simulink library "inp"  (R2021b)
settings: Solver=VariableStepAuto  StartTime=0.0  StopTime=10.0  RelTol=1e-3
undefined symbols (not defined in the file): C_TASK_5MS_S, FALSE, KINP_AcoreReadyToSlp_flg_ovrdflg, KINP_AcoreReadyToSlp_flg_ovrdval, KINP_AllowMovThd_OTA_enum_ovrdflg, KINP_AllowMovThd_OTA_enum_ovrdval, KINP_APSAngleTarget_Deg_ovrdflg, KINP_APSAngleTarget_Deg_ovrdval, KINP_APSDecReq_mps2_ovrdflg, KINP_APSDecReq_mps2_ovrdval, KINP_APSDecReqA_flg_ovrdflg, KINP_APSDecReqA_flg_ovrdval, KINP_APSDFLL_cm_ovrdflg, KINP_APSDFLL_cm_ovrdval, KINP_APSDFLR_cm_ovrdflg, KINP_APSDFLR_cm_ovrdval, KINP_APSDRLL_cm_ovrdflg, KINP_APSDRLL_cm_ovrdval, KINP_APSDRLR_cm_ovrdflg, KINP_APSDRLR_cm_ovrdval, KINP_APSExitCondition_enum_ovrdflg, KINP_APSExitCondition_enum_ovrdval, KINP_APSHWVer_enum_ovrdflg, KINP_APSHWVer_enum_ovrdval, KINP_APSProgressPCT_pct_ovrdflg, KINP_APSProgressPCT_pct_ovrdval, KINP_APSReq_enum_ovrdflg, KINP_APSReq_enum_ovrdval, KINP_APSRQDisplay_enum_ovrdflg, KINP_APSRQDisplay_enum_ovrdval, KINP_APSRqEPASCtrl_flg_ovrdflg, KINP_APSRqEPASCtrl_flg_ovrdval, KINP_APSShiftPosnReq_enum_ovrdval, KINP_APSShiftPosnReq_enum_ovrflg, KINP_APSSpeedCMD_kph_ovrdval, KINP_APSSpeedCMD_kph_ovrflg, KINP_APSStaSystem_enum_ovrdflg, KINP_APSStaSystem_enum_ovrdval, KINP_APSSWVer_enum_ovrdflg, KINP_APSSWVer_enum_ovrdval, KINP_APSVMCReqA_flg_ovrdval, KINP_APSVMCReqA_flg_ovrflg, KINP_APSVRqEPASCtrl_flg_ovrdflg, KINP_APSVRqEPASCtrl_flg_ovrdval, KINP_AuxBattVolmV_mV_ovrdflg, KINP_AuxBattVolmV_mV_ovrdval, KINP_CAASSta_enum_ovrdflg, KINP_CAASSta_enum_ovrdval, KINP_CAASVMCReqA_flg_ovrdval, KINP_CAASVMCReqA_flg_ovrflg, KINP_Chime_enum_ovrdflg, KINP_Chime_enum_ovrdval, KINP_ClearDTCcmd_flg_ovrdflg, KINP_ClearDTCcmd_flg_ovrdval, KINP_EvccAplusPwrUpReq_flg_ovrdflg, KINP_EvccAplusPwrUpReq_flg_ovrdval, KINP_LFID_raw_ovrdval, KINP_LFID_raw_ovrflg, KINP_LRID_raw_ovrdval, KINP_MemOffsetAccX_raw16_ovrdflg ... (+118)
libraries: FVT_lib x595, hcu_lib x1
(part 20 of 27)

== system inp/INP/CAN3/SignalCheck/MCU_F2 ==
  BHAL_outputs : Inport
  inp_CanValid_bus : Inport  Port=2
  FrCoolanttempReq : FVT_lib/inp/can_signal_template  SystemSampleTime=-1  VariantActivationTime=update diagram  Latency=0  AutoFrameSizeCalculation=off
      link override defval: Value=KINP_FrCoolanttempReq_C_defval
      link override fftdec: Value=KINP_FrCoolanttempReq_C_fftdec
      link override fftinc: Value=KINP_FrCoolanttempReq_C_fftinc
      link override fftlim: Value=KINP_FrCoolanttempReq_C_fftlim
      link override invalid: Value=KINP_FrCoolanttempReq_C_invalid
      link override ovrdflg: Value=KINP_FrCoolanttempReq_C_ovrdflg
      link override ovrdval: Value=KINP_FrCoolanttempReq_C_ovrdval
      link override setvalid: Value=KINP_FrCoolanttempReq_C_setvalid
      link override srvcflg: Value=KINP_FrCoolanttempReq_C_srvcflg
      link override srvcval: Value=KINP_FrCoolanttempReq_C_srvcval
  FrEOPSpdSet : FVT_lib/inp/can_signal_template  SystemSampleTime=-1  VariantActivationTime=update diagram  Latency=0  AutoFrameSizeCalculation=off
      link override defval: Value=KINP_FrEOPSpdSet_rpm_defval
      link override fftdec: Value=KINP_FrEOPSpdSet_rpm_fftdec
      link override fftinc: Value=KINP_FrEOPSpdSet_rpm_fftinc
      link override fftlim: Value=KINP_FrEOPSpdSet_rpm_fftlim
      link override invalid: Value=KINP_FrEOPSpdSet_rpm_invalid
      link override ovrdflg: Value=KINP_FrEOPSpdSet_rpm_ovrdflg
      link override ovrdval: Value=KINP_FrEOPSpdSet_rpm_ovrdval
      link override setvalid: Value=KINP_FrEOPSpdSet_rpm_setvalid
      link override srvcflg: Value=KINP_FrEOPSpdSet_rpm_srvcflg
      link override srvcval: Value=KINP_FrEOPSpdSet_rpm_srvcval
  FrFailcode1 : FVT_lib/inp/can_signal_template  SystemSampleTime=-1  VariantActivationTime=update diagram  Latency=0  AutoFrameSizeCalculation=off
      link override defval: Value=KINP_FrFailcode1_enum_defval
      link override fftdec: Value=KINP_FrFailcode1_enum_fftdec
      link override fftinc: Value=KINP_FrFailcode1_enum_fftinc
      link override fftlim: Value=KINP_FrFailcode1_enum_fftlim
      link override invalid: Value=KINP_FrFailcode1_enum_invalid
      link override ovrdflg: Value=KINP_FrFailcode1_enum_ovrdflg
      link override ovrdval: Value=KINP_FrFailcode1_enum_ovrdval
      link override setvalid: Value=KINP_FrFailcode1_enum_setvalid
      link override srvcflg: Value=KINP_FrFailcode1_enum_srvcflg
      link override srvcval: Value=KINP_FrFailcode1_enum_srvcval
  FrFailcode2 : FVT_lib/inp/can_signal_template  SystemSampleTime=-1  VariantActivationTime=update diagram  Latency=0  AutoFrameSizeCalculation=off
      link override defval: Value=KINP_FrFailcode2_enum_defval
      link override fftdec: Value=KINP_FrFailcode2_enum_fftdec
      link override fftinc: Value=KINP_FrFailcode2_enum_fftinc
      link override fftlim: Value=KINP_FrFailcode2_enum_fftlim
      link override invalid: Value=KINP_FrFailcode2_enum_invalid
      link override ovrdflg: Value=KINP_FrFailcode2_enum_ovrdflg
      link override ovrdval: Value=KINP_FrFailcode2_enum_ovrdval
      link override setvalid: Value=KINP_FrFailcode2_enum_setvalid
      link override srvcflg: Value=KINP_FrFailcode2_enum_srvcflg
      link override srvcval: Value=KINP_FrFailcode2_enum_srvcval
  FrFailcodehistory1 : FVT_lib/inp/can_signal_template  SystemSampleTime=-1  VariantActivationTime=update diagram  Latency=0  AutoFrameSizeCalculation=off
      link override defval: Value=KINP_FrFailcodehistory1_enum_defval
      link override fftdec: Value=KINP_FrFailcodehistory1_enum_fftdec
      link override fftinc: Value=KINP_FrFailcodehistory1_enum_fftinc
      link override fftlim: Value=KINP_FrFailcodehistory1_enum_fftlim
      link override invalid: Value=KINP_FrFailcodehistory1_enum_invalid
      link override ovrdflg: Value=KINP_FrFailcodehistory1_enum_ovrdflg
      link override ovrdval: Value=KINP_FrFailcodehistory1_enum_ovrdval
      link override setvalid: Value=KINP_FrFailcodehistory1_enum_setvalid
      link override srvcflg: Value=KINP_FrFailcodehistory1_enum_srvcflg
      link override srvcval: Value=KINP_FrFailcodehistory1_enum_srvcval
  FrFailcodehistory2 : FVT_lib/inp/can_signal_template  SystemSampleTime=-1  VariantActivationTime=update diagram  Latency=0  AutoFrameSizeCalculation=off
      link override defval: Value=KINP_FrFailcodehistory2_enum_defval
      link override fftdec: Value=KINP_FrFailcodehistory2_enum_fftdec
      link override fftinc: Value=KINP_FrFailcodehistory2_enum_fftinc
      link override fftlim: Value=KINP_FrFailcodehistory2_enum_fftlim
      link override invalid: Value=KINP_FrFailcodehistory2_enum_invalid
      link override ovrdflg: Value=KINP_FrFailcodehistory2_enum_ovrdflg
      link override ovrdval: Value=KINP_FrFailcodehistory2_enum_ovrdval
      link override setvalid: Value=KINP_FrFailcodehistory2_enum_setvalid
      link override srvcflg: Value=KINP_FrFailcodehistory2_enum_srvcflg
      link override srvcval: Value=KINP_FrFailcodehistory2_enum_srvcval
  FrLLCTemp : FVT_lib/inp/can_signal_template  SystemSampleTime=-1  VariantActivationTime=update diagram  Latency=0  AutoFrameSizeCalculation=off
      link override defval: Value=KINP_FrLLCTemp_C_defval
      link override fftdec: Value=KINP_FrLLCTemp_C_fftdec
      link override fftinc: Value=KINP_FrLLCTemp_C_fftinc
      link override fftlim: Value=KINP_FrLLCTemp_C_fftlim
      link override invalid: Value=KINP_FrLLCTemp_C_invalid
      link override ovrdflg: Value=KINP_FrLLCTemp_C_ovrdflg
      link override ovrdval: Value=KINP_FrLLCTemp_C_ovrdval
      link override setvalid: Value=KINP_FrLLCTemp_C_setvalid
      link override srvcflg: Value=KINP_FrLLCTemp_C_srvcflg
      link override srvcval: Value=KINP_FrLLCTemp_C_srvcval
  FrLLCflowReq : FVT_lib/inp/can_signal_template  SystemSampleTime=-1  VariantActivationTime=update diagram  Latency=0  AutoFrameSizeCalculation=off
      link override defval: Value=KINP_FrLLCflowReq_Lpmin_defval
      link override fftdec: Value=KINP_FrLLCflowReq_Lpmin_fftdec
      link override fftinc: Value=KINP_FrLLCflowReq_Lpmin_fftinc
      link override fftlim: Value=KINP_FrLLCflowReq_Lpmin_fftlim
      link override invalid: Value=KINP_FrLLCflowReq_Lpmin_invalid
      link override ovrdflg: Value=KINP_FrLLCflowReq_Lpmin_ovrdflg
      link override ovrdval: Value=KINP_FrLLCflowReq_Lpmin_ovrdval
      link override setvalid: Value=KINP_FrLLCflowReq_Lpmin_setvalid
      link override srvcflg: Value=KINP_FrLLCflowReq_Lpmin_srvcflg
      link override srvcval: Value=KINP_FrLLCflowReq_Lpmin_srvcval
  FrMCUTempWarn : FVT_lib/inp/can_signal_template  SystemSampleTime=-1  VariantActivationTime=update diagram  Latency=0  AutoFrameSizeCalculation=off
      link override defval: Value=KINP_FrMCUTempWarn_enum_defval
      link override fftdec: Value=KINP_FrMCUTempWarn_enum_fftdec
      link override fftinc: Value=KINP_FrMCUTempWarn_enum_fftinc
      link override fftlim: Value=KINP_FrMCUTempWarn_enum_fftlim
      link override invalid: Value=KINP_FrMCUTempWarn_enum_invalid
      link override ovrdflg: Value=KINP_FrMCUTempWarn_enum_ovrdflg
      link override ovrdval: Value=KINP_FrMCUTempWarn_enum_ovrdval
      link override setvalid: Value=KINP_FrMCUTempWarn_enum_setvalid
      link override srvcflg: Value=KINP_FrMCUTempWarn_enum_srvcflg
      link override srvcval: Value=KINP_FrMCUTempWarn_enum_srvcval
  FrTMTempWarn : FVT_lib/inp/can_signal_template  SystemSampleTime=-1  VariantActivationTime=update diagram  Latency=0  AutoFrameSizeCalculation=off
      link override defval: Value=KINP_FrTMTempWarn_enum_defval
      link override fftdec: Value=KINP_FrTMTempWarn_enum_fftdec
      link override fftinc: Value=KINP_FrTMTempWarn_enum_fftinc
      link override fftlim: Value=KINP_FrTMTempWarn_enum_fftlim
      link override invalid: Value=KINP_FrTMTempWarn_enum_invalid
      link override ovrdflg: Value=KINP_FrTMTempWarn_enum_ovrdflg
      link override ovrdval: Value=KINP_FrTMTempWarn_enum_ovrdval
      link override setvalid: Value=KINP_FrTMTempWarn_enum_setvalid
      link override srvcflg: Value=KINP_FrTMTempWarn_enum_srvcflg
      link override srvcval: Value=KINP_FrTMTempWarn_enum_srvcval
  Terminator_{1..10} (10 alike) : Terminator
  True_VHAL_FrCoolanttempReq_C : Constant  Value=TRUE  OutDataTypeStr=boolean
  True_VHAL_FrEOPSpdSet_rpm : Constant  Value=TRUE  OutDataTypeStr=boolean
  True_VHAL_FrFailcode1_enum : Constant  Value=TRUE  OutDataTypeStr=boolean
  True_VHAL_FrFailcode2_enum : Constant  Value=TRUE  OutDataTypeStr=boolean
  True_VHAL_FrFailcodehistory1_enum : Constant  Value=TRUE  OutDataTypeStr=boolean
  True_VHAL_FrFailcodehistory2_enum : Constant  Value=TRUE  OutDataTypeStr=boolean
  True_VHAL_FrLLCTemp_C : Constant  Value=TRUE  OutDataTypeStr=boolean
  True_VHAL_FrLLCflowReq_Lpmin : Constant  Value=TRUE  OutDataTypeStr=boolean
  True_VHAL_FrMCUTempWarn_enum : Constant  Value=TRUE  OutDataTypeStr=boolean
  True_VHAL_FrTMTempWarn_enum : Constant  Value=TRUE  OutDataTypeStr=boolean
  slr1_{1..10} (10 alike) : BusSelector  OutputSignals=VINP_CANMsgValidMCUF2_flg
  slr_VHAL_FrCoolanttempReq_C : BusSelector  OutputSignals=VHAL_FrCoolanttempReq_C
  slr_VHAL_FrEOPSpdSet_rpm : BusSelector  OutputSignals=VHAL_FrEOPSpdSet_rpm
  slr_VHAL_FrFailcode1_enum : BusSelector  OutputSignals=VHAL_FrFailcode1_enum
  slr_VHAL_FrFailcode2_enum : BusSelector  OutputSignals=VHAL_FrFailcode2_enum
  slr_VHAL_FrFailcodehistory1_enum : BusSelector  OutputSignals=VHAL_FrFailcodehistory1_enum
  slr_VHAL_FrFailcodehistory2_enum : BusSelector  OutputSignals=VHAL_FrFailcodehistory2_enum
  slr_VHAL_FrLLCTemp_C : BusSelector  OutputSignals=VHAL_FrLLCTemp_C
  slr_VHAL_FrLLCflowReq_Lpmin : BusSelector  OutputSignals=VHAL_FrLLCflowReq_Lpmin
  slr_VHAL_FrMCUTempWarn_enum : BusSelector  OutputSignals=VHAL_FrMCUTempWarn_enum
  slr_VHAL_FrTMTempWarn_enum : BusSelector  OutputSignals=VHAL_FrTMTempWarn_enum
  VINP_FrCoolanttempReq_C : Outport
  VINP_FrEOPSpdSet_rpm : Outport  Port=2
  VINP_FrFailcode1_enum : Outport  Port=3
  VINP_FrFailcode2_enum : Outport  Port=4
  VINP_FrFailcodehistory1_enum : Outport  Port=5
  VINP_FrFailcodehistory2_enum : Outport  Port=6
  VINP_FrLLCTemp_C : Outport  Port=7
  VINP_FrLLCflowReq_Lpmin : Outport  Port=8
  VINP_FrMCUTempWarn_enum : Outport  Port=9
  VINP_FrTMTempWarn_enum : Outport  Port=10
  wires:
  BHAL_outputs/1 -> [BHAL_outputs]
  inp_CanValid_bus/1 -> [inp_CanValid_bus]
  [BHAL_outputs] -> slr_VHAL_FrCoolanttempReq_C/1
  slr_VHAL_FrCoolanttempReq_C/1 -> FrCoolanttempReq/1  "<VHAL_FrCoolanttempReq_C>"
  True_VHAL_FrCoolanttempReq_C/1 -> FrCoolanttempReq/2
  [inp_CanValid_bus] -> slr1_1/1
  slr1_1/1 -> FrCoolanttempReq/3  "<VINP_CANMsgValidMCUF2_flg>"
  FrCoolanttempReq/1 -> VINP_FrCoolanttempReq_C/1  "VINP_FrCoolanttempReq_C"
  FrCoolanttempReq/2 -> Terminator_1/1
  [BHAL_outputs] -> slr_VHAL_FrEOPSpdSet_rpm/1
  slr_VHAL_FrEOPSpdSet_rpm/1 -> FrEOPSpdSet/1  "<VHAL_FrEOPSpdSet_rpm>"
  True_VHAL_FrEOPSpdSet_rpm/1 -> FrEOPSpdSet/2
  [inp_CanValid_bus] -> slr1_2/1
  slr1_2/1 -> FrEOPSpdSet/3  "<VINP_CANMsgValidMCUF2_flg>"
  FrEOPSpdSet/1 -> VINP_FrEOPSpdSet_rpm/1  "VINP_FrEOPSpdSet_rpm"
  FrEOPSpdSet/2 -> Terminator_2/1
  [BHAL_outputs] -> slr_VHAL_FrFailcode1_enum/1
  slr_VHAL_FrFailcode1_enum/1 -> FrFailcode1/1  "<VHAL_FrFailcode1_enum>"
  True_VHAL_FrFailcode1_enum/1 -> FrFailcode1/2
  [inp_CanValid_bus] -> slr1_3/1
  slr1_3/1 -> FrFailcode1/3  "<VINP_CANMsgValidMCUF2_flg>"
  FrFailcode1/1 -> VINP_FrFailcode1_enum/1  "VINP_FrFailcode1_enum"
  FrFailcode1/2 -> Terminator_3/1
  [BHAL_outputs] -> slr_VHAL_FrFailcode2_enum/1
  slr_VHAL_FrFailcode2_enum/1 -> FrFailcode2/1  "<VHAL_FrFailcode2_enum>"
  True_VHAL_FrFailcode2_enum/1 -> FrFailcode2/2
  [inp_CanValid_bus] -> slr1_4/1
  slr1_4/1 -> FrFailcode2/3  "<VINP_CANMsgValidMCUF2_flg>"
  FrFailcode2/1 -> VINP_FrFailcode2_enum/1  "VINP_FrFailcode2_enum"
  FrFailcode2/2 -> Terminator_4/1
  [BHAL_outputs] -> slr_VHAL_FrFailcodehistory1_enum/1
  slr_VHAL_FrFailcodehistory1_enum/1 -> FrFailcodehistory1/1  "<VHAL_FrFailcodehistory1_enum>"
  True_VHAL_FrFailcodehistory1_enum/1 -> FrFailcodehistory1/2
  [inp_CanValid_bus] -> slr1_5/1
  slr1_5/1 -> FrFailcodehistory1/3  "<VINP_CANMsgValidMCUF2_flg>"
  FrFailcodehistory1/1 -> VINP_FrFailcodehistory1_enum/1  "VINP_FrFailcodehistory1_enum"
  FrFailcodehistory1/2 -> Terminator_5/1
  [BHAL_outputs] -> slr_VHAL_FrFailcodehistory2_enum/1
  slr_VHAL_FrFailcodehistory2_enum/1 -> FrFailcodehistory2/1  "<VHAL_FrFailcodehistory2_enum>"
  True_VHAL_FrFailcodehistory2_enum/1 -> FrFailcodehistory2/2
  [inp_CanValid_bus] -> slr1_6/1
  slr1_6/1 -> FrFailcodehistory2/3  "<VINP_CANMsgValidMCUF2_flg>"
  FrFailcodehistory2/1 -> VINP_FrFailcodehistory2_enum/1  "VINP_FrFailcodehistory2_enum"
  FrFailcodehistory2/2 -> Terminator_6/1
  [BHAL_outputs] -> slr_VHAL_FrLLCTemp_C/1
  slr_VHAL_FrLLCTemp_C/1 -> FrLLCTemp/1  "<VHAL_FrLLCTemp_C>"
  True_VHAL_FrLLCTemp_C/1 -> FrLLCTemp/2
  [inp_CanValid_bus] -> slr1_7/1
  slr1_7/1 -> FrLLCTemp/3  "<VINP_CANMsgValidMCUF2_flg>"
  FrLLCTemp/1 -> VINP_FrLLCTemp_C/1  "VINP_FrLLCTemp_C"
  FrLLCTemp/2 -> Terminator_7/1
  [BHAL_outputs] -> slr_VHAL_FrLLCflowReq_Lpmin/1
  slr_VHAL_FrLLCflowReq_Lpmin/1 -> FrLLCflowReq/1  "<VHAL_FrLLCflowReq_Lpmin>"
  True_VHAL_FrLLCflowReq_Lpmin/1 -> FrLLCflowReq/2
  [inp_CanValid_bus] -> slr1_8/1
  slr1_8/1 -> FrLLCflowReq/3  "<VINP_CANMsgValidMCUF2_flg>"
  FrLLCflowReq/1 -> VINP_FrLLCflowReq_Lpmin/1  "VINP_FrLLCflowReq_Lpmin"
  FrLLCflowReq/2 -> Terminator_8/1
  [BHAL_outputs] -> slr_VHAL_FrMCUTempWarn_enum/1
  slr_VHAL_FrMCUTempWarn_enum/1 -> FrMCUTempWarn/1  "<VHAL_FrMCUTempWarn_enum>"
  True_VHAL_FrMCUTempWarn_enum/1 -> FrMCUTempWarn/2
  [inp_CanValid_bus] -> slr1_9/1
  slr1_9/1 -> FrMCUTempWarn/3  "<VINP_CANMsgValidMCUF2_flg>"
  FrMCUTempWarn/1 -> VINP_FrMCUTempWarn_enum/1  "VINP_FrMCUTempWarn_enum"
  FrMCUTempWarn/2 -> Terminator_9/1
  [BHAL_outputs] -> slr_VHAL_FrTMTempWarn_enum/1
  slr_VHAL_FrTMTempWarn_enum/1 -> FrTMTempWarn/1  "<VHAL_FrTMTempWarn_enum>"
  True_VHAL_FrTMTempWarn_enum/1 -> FrTMTempWarn/2
  [inp_CanValid_bus] -> slr1_10/1
  slr1_10/1 -> FrTMTempWarn/3  "<VINP_CANMsgValidMCUF2_flg>"
  FrTMTempWarn/1 -> VINP_FrTMTempWarn_enum/1  "VINP_FrTMTempWarn_enum"
  FrTMTempWarn/2 -> Terminator_10/1
